simulink model "hvac_maborrelli_singapur_nzones_with_MPC_v3_manualdist_3"  (R2021a)
settings: Solver=ode45  StartTime=0.0  StopTime=Inf  FixedStep=2  RelTol=1e-3  EnableMultiTasking=on
values from neighbouring files (symbols this model uses):
  ci = [30;30;30;30;30;30;30;30]    [main.m]
  sampling_time = 60    [main.m]
undefined symbols (not defined in the file or in its folder): paramsnz, rl, up
libraries: simulink x2, rllib x1
settings Model: Creator=User  LastModifiedBy=Richi
settings SolverCC: AlgebraicLoopSolver=TrustRegion
settings DataIOCC: LimitDataPoints=on  SaveFormat=Array  SignalLoggingSaveFormat=ModelDataLogs
settings OptimizationCC: LifeSpan=inf
settings DebuggingCC: SolverPrmCheckMsg=warning  MultiTaskDSMMsg=warning  MultiTaskCondExecSysMsg=none  MultiTaskRateTransMsg=warning  StrictBusMsg=ErrorOnBusTreatedAsVector  SFUnexpectedBacktrackingDiag=warning  SFNoUnconditionalDefaultTransitionDiag=warning  SFExecutionAtInitializationDiag=none  SFMachineParentedDataDiag=warning  ArithmeticOperatorsInVariantConditions=warning
settings HardwareCC: ProdBitPerPointer=32  ProdBitPerSizeT=32  ProdBitPerPtrDiffT=32  ProdLargestAtomicFloat=None  ProdIntDivRoundTo=Undefined  ProdEndianess=Unspecified  ProdWordSize=32  ProdHWDeviceType=32-bit Generic
settings ModelReferenceCC: PropagateSignalLabelsOutOfModel=off
settings SFSimCC: SimUseLocalCustomCode=off  CustomCodeUndefinedFunction=UseInterfaceOnly
settings RTWCC: RTWUseLocalCustomCode=off
settings CodeAppCC: StateflowObjectComments=on
settings GRTTargetCC: TargetLangStandard=C89/C90 (ANSI)
settings ConfigComp: CovMetricSettings=dw  CovSaveCumulativeToWorkspaceVar=on  CovSaveSingleToWorkspaceVar=on  CovExternalEMLEnable=off

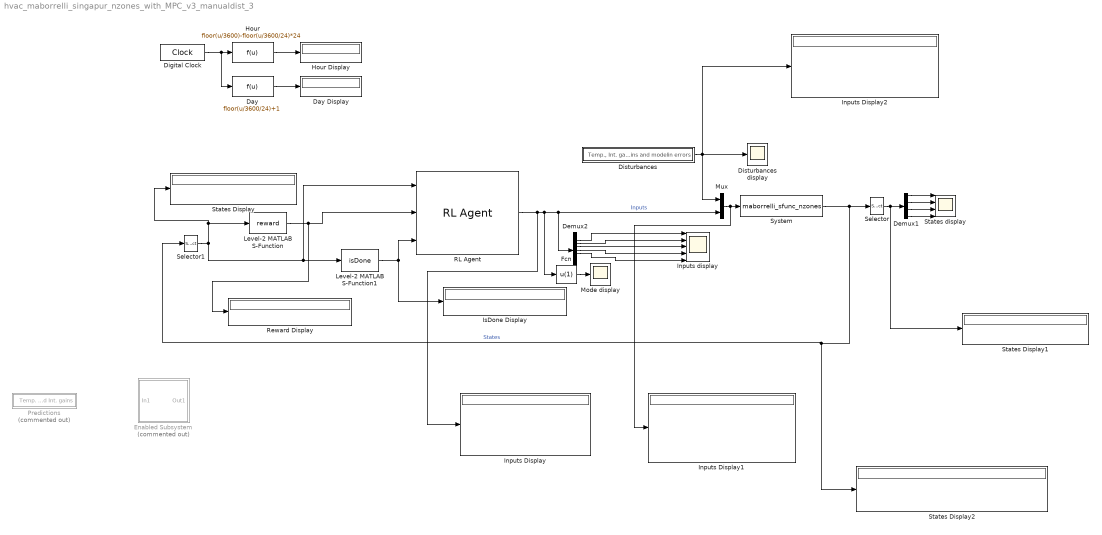
== system hvac_maborrelli_singapur_nzones_with_MPC_v3_manualdist_3 ==
  Day : Fcn  Expr=floor(u/3600/24)+1  SampleTime=1800
  Day Display : Display
  Demux1 : Demux
  Demux2 : Demux  Outputs=6
  Digital Clock : DigitalClock  SampleTime=60
  Disturbances : Subsystem  TreatAsAtomicUnit=on
  Disturbances display : Scope
  Enabled Subsystem : Subsystem  Commented=on  TreatAsAtomicUnit=on
  Fcn : Fcn  Expr=u(1)
  Hour : Fcn  Expr=floor(u/3600)-floor(u/3600/24)*24  SampleTime=1800
  Hour Display : Display
  Inputs Display : Display
  Inputs Display1 : Display
  Inputs Display2 : Display
  Inputs display : Scope  NumInputPorts=5
  IsDone Display : Display
  Level-2 MATLAB S-Function : M-S-Function  FunctionName=reward
  Level-2 MATLAB S-Function1 : M-S-Function  FunctionName=isDone
  Mode display : Scope
  Mux : Mux  Inputs=2
  Predictions : Subsystem  Commented=on  TreatAsAtomicUnit=on
  RL Agent : rllib/RL Agent  Agent=rl.util.PolicyInstance.get('hvac_maborrelli_singapur_nzones_with_MPC_v3_manualdist_3/RL Agent')  ExternalActionAsInput=off  ProvideCumRwd=off  TreatAsDirectFeedthrough=on
  Reward Display : Display
  Selector : Selector  InputPortWidth=8  IndexOptions=Index vector (dialog)  Indices=[1 2 3 4]  OutputSizes=1
  Selector1 : Selector  InputPortWidth=8  IndexOptions=Index vector (dialog)  Indices=[1 2 3 4]  OutputSizes=1
  States Display : Display
  States Display1 : Display
  States Display2 : Display
  States display : Scope  NumInputPorts=4
  System : S-Function  FunctionName=maborrelli_sfunc_nzones  Parameters=ci,paramsnz  SFunctionDeploymentMode=off  EnableBusSupport=off
  wires:
  Disturbances/1("Temp., Int. gains and modelin errors") -> Mux/1, Inputs Display2/1, Disturbances display/1
  Mux/1 -> Inputs Display1/1, System/1
  System/1 -> Selector/1, Selector1/1, States Display2/1  "States"
  RL Agent/1 -> Mux/2, Demux2/1, Fcn/1, Inputs Display/1  "Inputs"
  Fcn/1 -> Mode display/1
  Hour/1 -> Hour Display/1
  Digital Clock/1 -> Day/1, Hour/1
  Day/1 -> Day Display/1
  Selector/1 -> States Display1/1, Demux1/1
  Demux1/1 -> States display/1
  Demux1/2 -> States display/2
  Demux1/3 -> States display/3
  Demux1/4 -> States display/4
  Demux2/1 -> Inputs display/1
  Demux2/2 -> Inputs display/2
  Demux2/3 -> Inputs display/3
  Demux2/4 -> Inputs display/4
  Demux2/5 -> Inputs display/5
  Level-2 MATLAB S-Function1/1 -> RL Agent/3, IsDone Display/1
  Level-2 MATLAB S-Function/1 -> Reward Display/1, RL Agent/2
  Selector1/1 -> Level-2 MATLAB S-Function/1, States Display/1, RL Agent/1, Level-2 MATLAB S-Function1/1

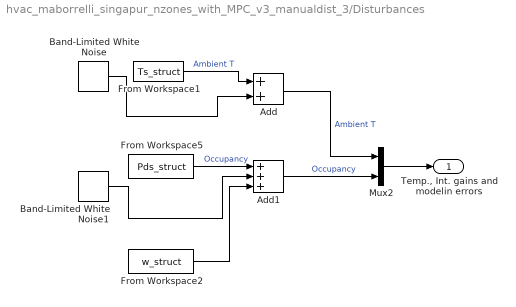
== system hvac_maborrelli_singapur_nzones_with_MPC_v3_manualdist_3/Disturbances ==
  Add : Sum
  Add1 : Sum  Inputs=+++
  Band-Limited White Noise : simulink/Sources/Band-Limited White Noise  Cov=0  Ts=sampling_time  seed=[23341]
  Band-Limited White Noise1 : simulink/Sources/Band-Limited White Noise  Cov=0  Ts=sampling_time  seed=[23341]
  From Workspace1 : FromWorkspace  VariableName=Ts_struct  OutDataTypeStr=double  SampleTime=sampling_time  ZeroCross=off
  From Workspace2 : FromWorkspace  VariableName=w_struct  OutDataTypeStr=double  SampleTime=sampling_time  ZeroCross=off
  From Workspace5 : FromWorkspace  VariableName=Pds_struct  OutDataTypeStr=double  SampleTime=sampling_time  ZeroCross=off
  Mux2 : Mux  Inputs=2
  "Temp., Int. gains and modelin errors" : Outport
  wires:
  Add1/1 -> Mux2/2  "Occupancy"
  From Workspace1/1 -> Add/1  "Ambient T"
  Band-Limited White Noise/1 -> Add/2
  Add/1 -> Mux2/1  "Ambient T"
  From Workspace5/1 -> Add1/1  "Occupancy"
  Band-Limited White Noise1/1 -> Add1/2
  From Workspace2/1 -> Add1/3
  Mux2/1 -> "Temp., Int. gains and modelin errors"/1

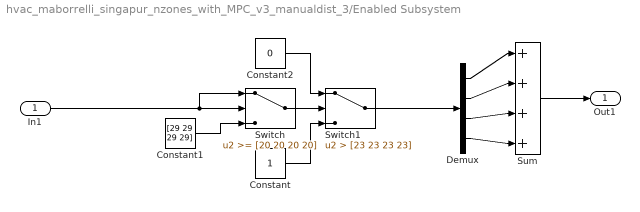
== system hvac_maborrelli_singapur_nzones_with_MPC_v3_manualdist_3/Enabled Subsystem ==
  In1 : Inport
  Constant : Constant
  Constant1 : Constant  Value=[29 29 29 29]
  Constant2 : Constant  Value=0
  Demux : Demux
  Sum : Sum  Inputs=|++++
  Switch : Switch  Threshold=[20 20 20 20]
  Switch1 : Switch  Criteria=u2 > Threshold  Threshold=[23 23 23 23]
  Out1 : Outport
  wires:
  In1/1 -> Switch/1, Switch/2
  Switch/1 -> Switch1/2
  Constant/1 -> Switch1/3
  Constant2/1 -> Switch1/1
  Constant1/1 -> Switch/3
  Switch1/1 -> Demux/1
  Demux/1 -> Sum/1
  Demux/2 -> Sum/2
  Demux/3 -> Sum/3
  Demux/4 -> Sum/4
  Sum/1 -> Out1/1

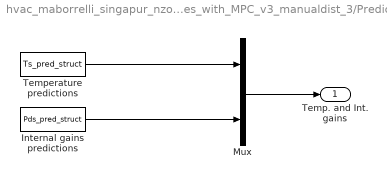
== system hvac_maborrelli_singapur_nzones_with_MPC_v3_manualdist_3/Predictions ==
  Internal gains predictions : FromWorkspace  VariableName=Pds_pred_struct  OutDataTypeStr=double  SampleTime=up.DeltaT  ZeroCross=off
  Mux : Mux  Inputs=2
  Temperature predictions : FromWorkspace  VariableName=Ts_pred_struct  OutDataTypeStr=double  SampleTime=up.DeltaT  ZeroCross=off
  Temp. and Int. gains : Outport
  wires:
  Internal gains predictions/1 -> Mux/2
  Temperature predictions/1 -> Mux/1
  Mux/1 -> Temp. and Int. gains/1
